simulink model "Woodward_v6_milestone"  (Simulink 7.8)
settings: Solver=ode5  StartTime=0.0  StopTime=inf  FixedStep=Ts  MaxStep=1e-3  RelTol=1e-3
PostLoadFcn:
  | Ts=50e-6;
InitFcn:
  | Ts=50e-6;
undefined symbols (not defined in the file): another_event_name, dfilt, DiscIntNeverNeededParam, fdesignblkfcn, gcbh, Gen_900kW_external_control, GenSet_900kW_07232015, HIL_GenSet, Left, my_event_name, ph, type, V
libraries: simulink x49, powerlib x33, rtio_opalrt_common x19, powerlib_extras x8, dspsigops x4, rtlab x3, cables_lib x3, simulink_extras x3, discretizing x2, rteventslib x2, dsparch4 x2, transformer_lib x1
(part 1 of 3)
settings Model: ARTEMISmethode_block_infos=$$__separator__$$  Creator=CH24070  LastModifiedBy=ma25949  BufferReuse=off
settings SolverCC: ZeroCrossAlgorithm=Adaptive
settings DataIOCC: ExternalInput=getinputstruct(op_snapshot1)  InitialState=getstatestruct(op_snapshot1)  LimitDataPoints=off  MaxDataPoints=90060  SignalLoggingSaveFormat=Dataset  SaveOutput=off  SignalLogging=off  DSMLogging=off  SaveTime=off  OutputSaveName=result
settings OptimizationCC: BlockReduction=off  OptimizeBlockIOStorage=off  BufferReuse=off  ExpressionFolding=off  LocalBlockOutputs=off
settings DebuggingCC: MaxConsecutiveZCsMsg=warning  IgnoredZcDiagnostic=none  SolverPrmCheckMsg=none  MultiTaskRateTransMsg=warning  FrameProcessingCompatibilityMsg=error  ModelReferenceExtraNoncontSigs=warning
settings ModelReferenceCC: UpdateModelReferenceTargets=IfOutOfDate
settings SFSimCC: SFSimEcho=off
settings CodeAppCC: CustomSymbolStrType=$N$R$M_T
settings GRTTargetCC: TargetFunctionLibrary=C89/C90 (ANSI)
settings CustomProperty: DataType=string  Value=0

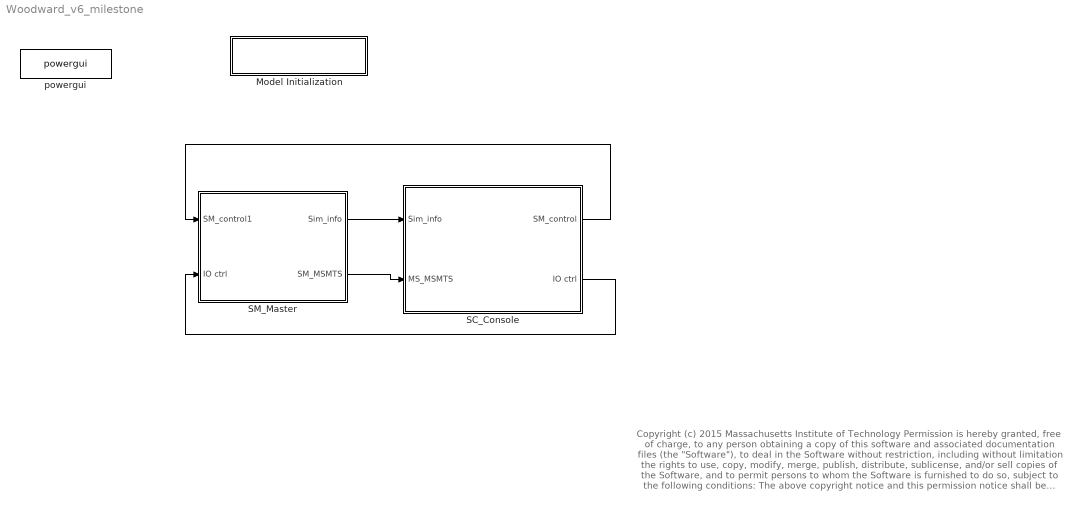
== system Woodward_v6_milestone ==
  note: Copyright (c) 2015 Massachusetts Institute of Technology
      | Permission is hereby granted, free of charge, to any person obtaining a copy of this software and associated documentation files (the "Software"), to deal in the Software without restriction, including without limitation the rights to use, copy, modify, merge, publish, distribute, sublicense, and/or sell copies of the Software, and to permit persons to whom the Software is furnished to do so, subject to the following conditions:
      |
      | The above copyright notice and this permission notice shall be included in all copies or substantial portions of the Software.
      |
      | THE SOFTWARE IS PROVIDED "AS IS", WITHOUT WARRANTY OF ANY KIND, EXPRESS OR IMPLIED, INCLUDING BUT NOT LIMITED TO THE WARRANTIES OF MERCHANTABILITY, FITNESS FOR A PARTICULAR PURPOSE AND NONINFRINGEMENT. IN NO EVENT SHALL THE AUTHORS OR COPYRIGHT HOLDERS BE LIABLE FOR ANY CLAIM,
      | DAMAGES OR OTHER LIABILITY, WHETHER IN AN ACTION OF CONTRACT, TORT OR OTHERWISE, ARISING FROM, OUT OF OR IN CONNECTION WITH THE SOFTWARE OR THE USE OR OTHER DEALINGS IN THE SOFTWARE.
  Model Initialization : Subsystem  AncestorBlock=artemis/Tools /Misc/Model Initialization  mask(Model Functions){InitFcnX=Ts=50e-6;, prel=off, posl=on, inif=on, strf=off}
      mask prompts: InitFcnX "Initialisation"; prel "Preload Function"; posl "PostLoad Function"; inif "InitFcn"; strf "StartFcn"
      mask init:
      | currentBlock = gcb;
      | root = bdroot(currentBlock);
      | 
      | if ~strcmp(get_param(root,'BlockDiagramType'),'library')
      |     if prel==1
      |         set_param(root, 'PreLoadFcn', InitFcnX);
      |     else
      |         set_param(root, 'PreLoadFcn', '');
      |     end
      |     if inif==1
      |         set_param(root, 'InitFcn', InitFcnX);
      |     else
      |         set_param(root, 'InitFcn', '');
      |     end
      |     if strf==1
      |         set_param(root, 'StartFcn', InitFcnX);
      |     else
      |         set_param(root, 'StartFcn', '');
      |     end
      |     if posl==1
      |         set_param(root, 'PostLoadFcn', InitFcnX);
      |     else
      |         set_param(root, 'PostLoadFcn', '');
      |     end
      | end
      | 
      | pos = get_param(currentBlock, 'Position');
      | width = pos(3) - pos(1); height = pos(4) - pos(2);
      | txt = [ upper(root) '\n' '- InitFcn. . . . . '  get_param(root, 'InitFcn') ];
      settings: CopyFcn=set_param(gcb,'LinkStatus','inactive')
      mask Display: text(5, height*0.5, txt, 'horizontalAlignment', 'left', 'verticalAlignment', 'middle') ;
  SC_Console : Subsystem
  SM_Master : Subsystem
  powergui : powerlib/powergui  Priority=2  SimulationMode=Discrete  SolverType=Tustin  SampleTime=Ts  frequency=60  SPID=off  DisableSnubberDevices=off  DisableRonSwitches=off  DisableVfSwitches=off  SwTol=0  Interpol=off  DisplayEquations=off  FunctionMessages=off  frequencyindice=0  Pbase=100e6  ErrMax=1e-4  Iterations=50  UnitsV=kV  UnitsW=MW  echomessages=off  HookPort=off  EnableUseOfTLC=off  x0status=blocks  RestoreLinks=warning  ResistiveCurrentMeasurement=off  Frange=logspace(0,3,50)  Ylog=off  Xlog=off  ShowGrid=off  save=off  variable=ZData  structure=0  ZoomFFT=on  StartTime=0.0  cycles=2  DisplayStyle=off  fundamental=60  FreqAxis=off  MaxFrequency=1000  frequencyindicesteady=1  RmsSteady=1  display=off  Ts=0  methode=off
  wires:
  SM_Master/1(Sim_info) -> SC_Console/1(Sim_info)
  SM_Master/2(SM_MSMTS) -> SC_Console/2(MS_MSMTS)
  SC_Console/1(SM_control) -> SM_Master/1(SM_control1)
  SC_Console/2(IO ctrl) -> SM_Master/2(IO ctrl)

== system Woodward_v6_milestone/Model Initialization ==

== system Woodward_v6_milestone/SC_Console ==
  note: Tcomputation
      | Ttotal
      | Idle
      | Overruns
  note: The 'Overruns' value should remain at 0.
      | The 'Ttotal' value should be equal to the
      | model Fixed-Step size.
  note: Ctrl Error
  Sim_info : Inport
  MS_MSMTS : Inport  Port=2
  B001 : Subsystem
  B031 : Subsystem
  Bus Creator : BusCreator  Inputs=2
  Bus Selector : BusSelector  OutputSignals=B031_PRM,B021_PRM,GEN_900kW_PRM,B012_PRM,B001_PRM,GEN_3p5MW_PRM,signal7,signal8,signal9,Load
  Demux5 : Demux  Outputs=[1 8 4]
  GEN900KW : Subsystem
  Gen_900kW_B001 : Subsystem  AncestorBlock=HIL_GenSet/Gen_900kW_external_control
  Load : Subsystem
  OpComm : rtlab/OpComm  nbport=2  groupe_acq=1  subsys_rate=0  st=0  Synchronization=on  Interpolation=on  Threshold=1.0  Missed_Data=off  Sim_Time=off  Samples=off  dynSigOut=off  from_console=0  warning_done=off  writeOpCommFile=off  Offset=off
  Status Codes : Display
      settings: Decimation=100
  TimingValues : Display
      settings: Decimation=100
  Woodward 900kW : Subsystem
  SM_control : Outport
  IO ctrl : Outport  Port=2
  wires:
  Sim_info/1 -> OpComm/1
  MS_MSMTS/1 -> OpComm/2
  Gen_900kW_B001/1(S) -> Bus Creator/1  "Gen_B001"
  Bus Creator/1 -> SM_control/1
  OpComm/2 -> Bus Selector/1
  Bus Selector/1 -> B031/1(S)  "<B031_PRM>"
  Bus Selector/3 -> GEN900KW/1(S)  "<GEN_900kW_PRM>"
  Bus Selector/5 -> B001/1(S)  "<B001_PRM>"
  Demux5/3 -> TimingValues/1
  OpComm/1 -> Demux5/1
  Demux5/1 -> Status Codes/1
  Bus Selector/8 -> Woodward 900kW/1(Gen_Primary)  "<signal8>"
  Bus Selector/9 -> Woodward 900kW/2(DIn_Ch00_31)  "<signal9>"
  Bus Selector/10 -> Load/1(S)  "<Load>"
  Woodward 900kW/1(Out1) -> IO ctrl/1

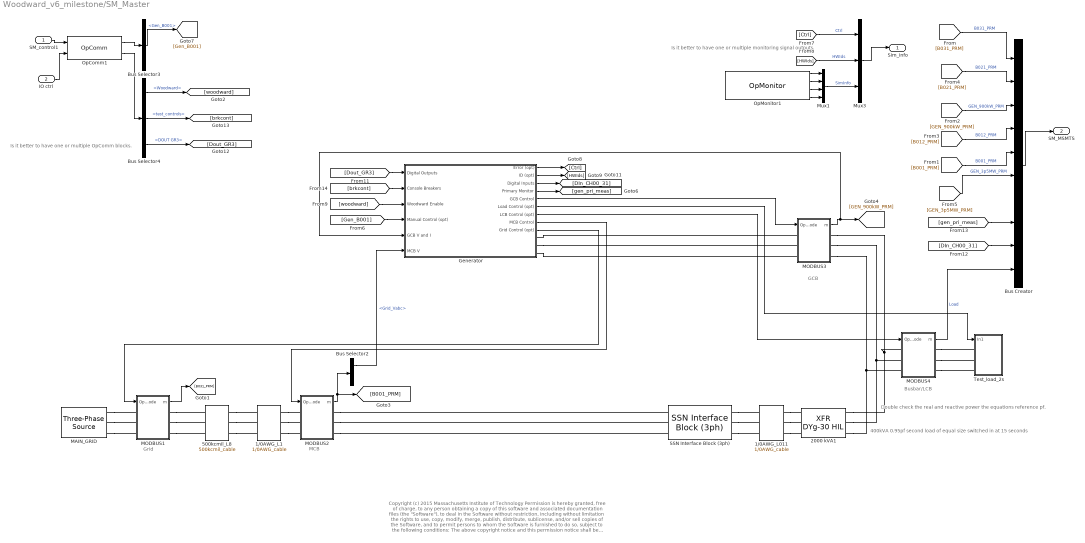
== system Woodward_v6_milestone/SM_Master ==
  note: Double check the real and reactive power
      | the equations reference pf.
  note: 400kVA 0.95pf
      | second load of equal size
      | switched in at 15 seconds
  note: Is it better to have one
      | or multiple OpComm blocks.
  note: Is it better to have one or multiple
      | monitoring signal outputs.
  note: GCB
  note: Busbar/LCB
  note: MCB
  note: Grid
  note: Copyright (c) 2015 Massachusetts Institute of Technology
      | Permission is hereby granted, free of charge, to any person obtaining a copy of this software and associated documentation files (the "Software"), to deal in the Software without restriction, including without limitation the rights to use, copy, modify, merge, publish, distribute, sublicense, and/or sell copies of the Software, and to permit persons to whom the Software is furnished to do so, subject to the following conditions:
      |
      | The above copyright notice and this permission notice shall be included in all copies or substantial portions of the Software.
      |
      | THE SOFTWARE IS PROVIDED "AS IS", WITHOUT WARRANTY OF ANY KIND, EXPRESS OR IMPLIED, INCLUDING BUT NOT LIMITED TO THE WARRANTIES OF MERCHANTABILITY, FITNESS FOR A PARTICULAR PURPOSE AND NONINFRINGEMENT. IN NO EVENT SHALL THE AUTHORS OR COPYRIGHT HOLDERS BE LIABLE FOR ANY CLAIM,
      | DAMAGES OR OTHER LIABILITY, WHETHER IN AN ACTION OF CONTRACT, TORT OR OTHERWISE, ARISING FROM, OUT OF OR IN CONNECTION WITH THE SOFTWARE OR THE USE OR OTHER DEALINGS IN THE SOFTWARE.
  SM_control1 : Inport
  IO ctrl : Inport  Port=2
  1/0AWG_L011 : cables_lib/1//0AWG_cable  length=1000  par_sets=1
  1/0AWG_L1 : cables_lib/1//0AWG_cable  length=1  par_sets=1
  2000 kVA1 : transformer_lib/XFR DYg-30 HIL  Rating=2000  Vp=13800  Vs=480  Z=5.75  XR=5.7
  500kcmil_L8 : cables_lib/500kcmil_cable  length=1  par_sets=1
  Bus Creator : BusCreator  Inputs=10
  Bus Selector2 : BusSelector  OutputSignals=sel_787.Grid_Vabc,sel_787.Iabc
  Bus Selector3 : BusSelector  OutputSignals=Gen_B001
  Bus Selector4 : BusSelector  OutputSignals=Woodward,test_controls,DOUT GR3
  Generator : Subsystem
  MAIN_GRID : powerlib/Electrical Sources/Three-Phase Source  Voltage=13800  PhaseAngle=0  Frequency=60  InternalConnection=Yg  SpecifyImpedance=on  Resistance=0.8929  Inductance=16.58e-3  ShortCircuitLevel=375e6  BaseVoltage=13800  XRratio=7.9  BusType=swing  Pref=0  Qref=0  Qmin=-inf  Qmax=inf
  MODBUS1 : Subsystem  mask(Protection and Metering){IOC=15E3, TOC=1800, Ts=Ts, VRMSLL=13800, I_nom=200}
      mask prompts: IOC "IOC setting [A]"; TOC "TOC setting [A]"; Ts "Sampling Time [Sec]"; VRMSLL "Nominal Voltage [VRMSLL]"; I_nom "Continous Current [A]"
      mask help:
      | This block simulates the behavior of selected relay functions as well as metering equipment.
      | The block is intended to communicate with a microgrid controller providing it measurements, and switching controls.
      mask Help:
      | This block simulates the behavior of selected relay functions as well as metering equipment (60 Hz - only).
      | The block is intended to communicate with a microgrid controller providing it measurements, and switching controls.
      | 
      | The input parameters are:
      | 0) Ts:  Sampling time [Seconds]
      | 1) State: 0 for relay logic mode, 1 to close the controlled breaker/switch,
      | and 2 to open the controlled breaker/switch
      | 2) TOC: Time-inverse overcurrent setting [Amperes]
      | 3) IOC: Instantaneous overcurrent setting [Amperes]
      | 
      | Metered parameters are:
      | 0) Status (0-closed, 1-open)
      | 1) Instantaneous voltage (abc)
      | 2) Instantaneous current (abc)
  MODBUS2 : Subsystem  mask(Protection and Metering){IOC=15E3, TOC=1800, Ts=Ts, VRMSLL=13800, I_nom=200}
      mask prompts: IOC "IOC setting [A]"; TOC "TOC setting [A]"; Ts "Sampling Time [Sec]"; VRMSLL "Nominal Voltage [VRMSLL]"; I_nom "Continous Current [A]"
      mask help:
      | This block simulates the behavior of selected relay functions as well as metering equipment.
      | The block is intended to communicate with a microgrid controller providing it measurements, and switching controls.
      mask Help:
      | This block simulates the behavior of selected relay functions as well as metering equipment (60 Hz - only).
      | The block is intended to communicate with a microgrid controller providing it measurements, and switching controls.
      | 
      | The input parameters are:
      | 0) Ts:  Sampling time [Seconds]
      | 1) State: 0 for relay logic mode, 1 to close the controlled breaker/switch,
      | and 2 to open the controlled breaker/switch
      | 2) TOC: Time-inverse overcurrent setting [Amperes]
      | 3) IOC: Instantaneous overcurrent setting [Amperes]
      | 
      | Metered parameters are:
      | 0) Status (0-closed, 1-open)
      | 1) Instantaneous voltage (abc)
      | 2) Instantaneous current (abc)
  MODBUS3 : Subsystem  mask(Protection and Metering){IOC=15E3, TOC=1800, Ts=Ts, VRMSLL=460, I_nom=200}
      mask prompts: IOC "IOC setting [A]"; TOC "TOC setting [A]"; Ts "Sampling Time [Sec]"; VRMSLL "Nominal Voltage [VRMSLL]"; I_nom "Continous Current [A]"
      mask help:
      | This block simulates the behavior of selected relay functions as well as metering equipment.
      | The block is intended to communicate with a microgrid controller providing it measurements, and switching controls.
      mask Help:
      | This block simulates the behavior of selected relay functions as well as metering equipment (60 Hz - only).
      | The block is intended to communicate with a microgrid controller providing it measurements, and switching controls.
      | 
      | The input parameters are:
      | 0) Ts:  Sampling time [Seconds]
      | 1) State: 0 for relay logic mode, 1 to close the controlled breaker/switch,
      | and 2 to open the controlled breaker/switch
      | 2) TOC: Time-inverse overcurrent setting [Amperes]
      | 3) IOC: Instantaneous overcurrent setting [Amperes]
      | 
      | Metered parameters are:
      | 0) Status (0-closed, 1-open)
      | 1) Instantaneous voltage (abc)
      | 2) Instantaneous current (abc)
  MODBUS4 : Subsystem  mask(Protection and Metering){IOC=15E3, TOC=1800, Ts=Ts, VRMSLL=460, I_nom=200}
      mask prompts: IOC "IOC setting [A]"; TOC "TOC setting [A]"; Ts "Sampling Time [Sec]"; VRMSLL "Nominal Voltage [VRMSLL]"; I_nom "Continous Current [A]"
      mask help:
      | This block simulates the behavior of selected relay functions as well as metering equipment.
      | The block is intended to communicate with a microgrid controller providing it measurements, and switching controls.
      mask Help:
      | This block simulates the behavior of selected relay functions as well as metering equipment (60 Hz - only).
      | The block is intended to communicate with a microgrid controller providing it measurements, and switching controls.
      | 
      | The input parameters are:
      | 0) Ts:  Sampling time [Seconds]
      | 1) State: 0 for relay logic mode, 1 to close the controlled breaker/switch,
      | and 2 to open the controlled breaker/switch
      | 2) TOC: Time-inverse overcurrent setting [Amperes]
      | 3) IOC: Instantaneous overcurrent setting [Amperes]
      | 
      | Metered parameters are:
      | 0) Status (0-closed, 1-open)
      | 1) Instantaneous voltage (abc)
      | 2) Instantaneous current (abc)
  Mux1 : Mux
  Mux3 : Mux  Inputs=[1 8 4]
  OpComm1 : rtlab/OpComm  nbport=2  groupe_acq=1  subsys_rate=0  st=0  Synchronization=on  Interpolation=on  Threshold=1.0  Missed_Data=off  Sim_Time=off  Samples=off  dynSigOut=off  from_console=1  warning_done=off  writeOpCommFile=off  Offset=off
  OpMonitor1 : rtlab/Monitoring/OpMonitor  compute_time=on  real_step=on  idle_time=on  nb_overruns=on  user_time=off  user_name=my_event_name,another_event_name
  SSN Interface Block (3ph) : ssn_lib/SSN Interface Block (3ph)  nb_phase=3  nb_port=2  p1_type=V-type(Left)  p2_type=V-type (Right)  p3_type=V-type(Left)  p4_type=V-type(Left)  p5_type=V-type(Left)  p6_type=V-type(Left)  p7_type=V-type(Left)  p8_type=V-type(Left)  p9_type=V-type(Left)  p10_type=V-type(Left)  p11_type=V-type(Left)  p12_type=V-type(Left)  p13_type=V-type(Left)  p14_type=V-type(Left)  p15_type=V-type(Left)  p16_type=V-type(Left)  I_port_shunt_resistance=1e9
  Test_load_2s : Subsystem  mask{v=460, kVA=400, pf=0.95}
      mask prompts: v "VRMSLL"
  Sim_info : Outport
  SM_MSMTS : Outport  Port=2
  wires:
  [B031_PRM] -> Bus Creator/1  "B031_PRM"
  [GEN_900kW_PRM] -> Bus Creator/3  "GEN_900kW_PRM"
  [B012_PRM] -> Bus Creator/4  "B012_PRM"
  [B021_PRM] -> Bus Creator/2  "B021_PRM"
  Bus Creator/1 -> SM_MSMTS/1
  [B001_PRM] -> Bus Creator/5  "B001_PRM"
  [GEN_3p5MW_PRM] -> Bus Creator/6  "GEN_3p5MW_PRM"
  [DIn_CH00_31] -> Bus Creator/9
  SM_control1/1 -> OpComm1/1
  OpComm1/1 -> Bus Selector3/1
  Bus Selector3/1 -> [Gen_B001]  "<Gen_B001>"
  OpComm1/2 -> Bus Selector4/1
  Bus Selector4/1 -> [woodward]  "<Woodward>"
  IO ctrl/1 -> OpComm1/2
  Bus Selector4/3 -> [Dout_GR3]  "<DOUT GR3>"
  OpMonitor1/1 -> Mux1/1
  OpMonitor1/2 -> Mux1/2
  OpMonitor1/3 -> Mux1/3
  OpMonitor1/4 -> Mux1/4
  Mux1/1 -> Mux3/3  "SimInfo"
  [Ctrl] -> Mux3/1  "Ctrl"
  [HWIds] -> Mux3/2  "HWIds"
  Mux3/1 -> Sim_info/1
  [gen_pri_meas] -> Bus Creator/8
  Bus Selector4/2 -> [brkcont]  "<test_controls>"
  MODBUS1/1(m) -> [B031_PRM]
  MODBUS2/1(m) -> Bus Selector2/1, [B001_PRM]
  MODBUS3/1(m) -> [GEN_900kW_PRM], Generator/5(GCB V and I)
  MODBUS4/1(m) -> Bus Creator/10  "Load"
  [Dout_GR3] -> Generator/1(Digital Outputs)
  [brkcont] -> Generator/2(Console Breakers)
  Generator/4(Primary Monitor) -> [gen_pri_meas]
  Generator/1(Error (opt)) -> [Ctrl]
  Generator/2(ID (opt)) -> [HWIds]
  Generator/3(Digital Inputs) -> [DIn_CH00_31]
  Bus Selector2/1 -> Generator/6(MCB V)  "<Grid_Vabc>"
  [Gen_B001] -> Generator/4(Manual Control (opt))
  [woodward] -> Generator/3(Woodward Enable)
  Generator/5(GCB Control) -> MODBUS3/1(Op_Mode)
  Generator/6(Load Control (opt)) -> Test_load_2s/1(In1)
  Generator/7(LCB Control (opt)) -> MODBUS4/1(Op_Mode)
  Generator/8(MCB Control) -> MODBUS2/1(Op_Mode)
  Generator/9(Grid Control (opt)) -> MODBUS1/1(Op_Mode)
  connections:
  1/0AWG_L011/RConn1 -- 2000 kVA1/LConn1
  1/0AWG_L011/RConn2 -- 2000 kVA1/LConn2
  1/0AWG_L011/RConn3 -- 2000 kVA1/LConn3
  SSN Interface Block (3ph)/RConn3 -- 1/0AWG_L011/LConn3
  SSN Interface Block (3ph)/RConn2 -- 1/0AWG_L011/LConn2
  SSN Interface Block (3ph)/RConn1 -- 1/0AWG_L011/LConn1
  MODBUS4/RConn3 -- Test_load_2s/LConn3
  MODBUS4/RConn2 -- Test_load_2s/LConn2
  MODBUS4/RConn1 -- Test_load_2s/LConn1
  2000 kVA1/RConn3 -- MODBUS4/LConn3 -- MODBUS3/RConn3
  2000 kVA1/RConn2 -- MODBUS4/LConn2 -- MODBUS3/RConn2
  2000 kVA1/RConn1 -- MODBUS4/LConn1 -- MODBUS3/RConn1
  MODBUS1/RConn3 -- 500kcmil_L8/LConn3
  MODBUS1/RConn2 -- 500kcmil_L8/LConn2
  MODBUS1/RConn1 -- 500kcmil_L8/LConn1
  MAIN_GRID/RConn3 -- MODBUS1/LConn3
  MAIN_GRID/RConn2 -- MODBUS1/LConn2
  MAIN_GRID/RConn1 -- MODBUS1/LConn1
  Generator/RConn3 -- MODBUS3/LConn3
  Generator/RConn2 -- MODBUS3/LConn2
  Generator/RConn1 -- MODBUS3/LConn1
  MODBUS2/RConn3 -- SSN Interface Block (3ph)/LConn3
  MODBUS2/RConn2 -- SSN Interface Block (3ph)/LConn2
  MODBUS2/RConn1 -- SSN Interface Block (3ph)/LConn1
  500kcmil_L8/RConn1 -- 1/0AWG_L1/LConn1
  500kcmil_L8/RConn2 -- 1/0AWG_L1/LConn2
  500kcmil_L8/RConn3 -- 1/0AWG_L1/LConn3
  1/0AWG_L1/RConn1 -- MODBUS2/LConn1
  1/0AWG_L1/RConn2 -- MODBUS2/LConn2
  1/0AWG_L1/RConn3 -- MODBUS2/LConn3

== system Woodward_v6_milestone/SC_Console/B001 ==
  S : Inport
  Bus Selector : BusSelector  OutputSignals=Grid_Status,sel_787.Grid_Vabc,sel_787.Iabc,sel_787.Grid_P,sel_787.Grid_Q
  Scope Mains : Scope  NumInputPorts=5
      settings: TimeRange=20  YMin=0~-15000~-500~-1e+006~-1e+006  YMax=1~15000~500~1e+006~1e+006  SaveName=ScopeData6
  wires:
  S/1 -> Bus Selector/1
  Bus Selector/1 -> Scope Mains/1  "<Grid_Status>"
  Bus Selector/2 -> Scope Mains/2  "<Grid_Vabc>"
  Bus Selector/3 -> Scope Mains/3  "<Iabc>"
  Bus Selector/4 -> Scope Mains/4  "<Grid_P>"
  Bus Selector/5 -> Scope Mains/5  "<Grid_Q>"

== system Woodward_v6_milestone/SC_Console/B031 ==
  S : Inport
  Bus Selector : BusSelector  OutputSignals=Grid_Status,sel_787.Grid_Vabc,sel_787.Iabc,sel_787.Grid_P,sel_787.Grid_Q
  Scope Grid : Scope  NumInputPorts=5
      settings: TimeRange=20  YMin=0~-20000~-20000~-1e+006~-1e+006  YMax=1~20000~20000~1e+006~1e+006
  wires:
  Bus Selector/1 -> Scope Grid/1  "<Grid_Status>"
  Bus Selector/2 -> Scope Grid/2  "<Grid_Vabc>"
  Bus Selector/3 -> Scope Grid/3  "<Iabc>"
  Bus Selector/4 -> Scope Grid/4  "<Grid_P>"
  Bus Selector/5 -> Scope Grid/5  "<Grid_Q>"
  S/1 -> Bus Selector/1

== system Woodward_v6_milestone/SC_Console/GEN900KW ==
  S : Inport
  Bus Selector : BusSelector  OutputSignals=Grid_Status,sel_787.Grid_Vabc,sel_787.Iabc,sel_787.Grid_P,sel_787.Grid_Q
  Scope Gen : Scope  NumInputPorts=5
      settings: TimeRange=60  YMin=0~-700~-2000~-1000000~-1000000  YMax=1~700~2000~1000000~1000000  SaveName=ScopeData5
  wires:
  S/1 -> Bus Selector/1
  Bus Selector/1 -> Scope Gen/1  "<Grid_Status>"
  Bus Selector/2 -> Scope Gen/2  "<Grid_Vabc>"
  Bus Selector/3 -> Scope Gen/3  "<Iabc>"
  Bus Selector/4 -> Scope Gen/4  "<Grid_P>"
  Bus Selector/5 -> Scope Gen/5  "<Grid_Q>"

== system Woodward_v6_milestone/SC_Console/Gen_900kW_B001 ==
  1 - PQ 2 - PV 3 - VF : Constant  Value=3
  Bus Creator : BusCreator  Inputs=6
  DONOTCHANGE : Constant
  Enable = 1 Disable = 0 : Constant  Value=0
  F : simulink/Math Operations/Slider Gain  low=0.97  gain=1  high=1.03
  P : simulink/Math Operations/Slider Gain  low=0  gain=0.8  high=1.1
  Q : simulink/Math Operations/Slider Gain  low=0.01  gain=0.2  high=0.4
  V : simulink/Math Operations/Slider Gain  low=0.9  gain=1  high=1.1
  S : Outport
  wires:
  DONOTCHANGE/1 -> P/1, Q/1, V/1, F/1
  Bus Creator/1 -> S/1
  P/1 -> Bus Creator/1  "P"
  Q/1 -> Bus Creator/2  "Q"
  V/1 -> Bus Creator/3  "V"
  F/1 -> Bus Creator/4  "F"
  1 - PQ 2 - PV 3 - VF/1 -> Bus Creator/5  "Mode"
  Enable = 1 Disable = 0/1 -> Bus Creator/6  "Enable"

== system Woodward_v6_milestone/SC_Console/Load ==
  S : Inport
  Bus Selector : BusSelector  OutputSignals=Grid_Status,sel_787.Grid_Vabc,sel_787.Iabc,sel_787.Grid_P,sel_787.Grid_Q
  Scope Load : Scope  NumInputPorts=5
      settings: TimeRange=20  YMin=0~-600~-2000~-1e+006~-1e+006  YMax=1~600~2000~1e+006~1e+006
  wires:
  Bus Selector/1 -> Scope Load/1  "<Grid_Status>"
  Bus Selector/2 -> Scope Load/2  "<Grid_Vabc>"
  Bus Selector/3 -> Scope Load/3  "<Iabc>"
  Bus Selector/4 -> Scope Load/4  "<Grid_P>"
  Bus Selector/5 -> Scope Load/5  "<Grid_Q>"
  S/1 -> Bus Selector/1

== system Woodward_v6_milestone/SC_Console/Woodward 900kW ==
  note: Op_Mode:
      | 0 = Relay Functions
      | 1 = Close Breaker
      | 2 = Open Breaker
  note: This corresponds to
      | the DIO Enable MCB
  Gen_Primary : Inport
  DIn_Ch00_31 : Inport  Port=2
  16Din/16Dout GR3 : Subsystem
  16PWMIn/16PWMout GR3 : Subsystem
  16TSDIn/16 TSDOut GR3 : Subsystem
  Brk1 Grid : Constant  Value=2
  Brk2 MCB : Constant  Value=2
  Brk3 GCB : Constant
  Brk4 Load : Constant  Value=2
  Bus Creator1 : BusCreator  Inputs=3
  Bus Creator2 : BusCreator  Inputs=3
  Bus Creator3 : BusCreator  Inputs=9
  Bus Selector1 : BusSelector  OutputSignals=Pm,Vf,Vt,w
  Scope_Primary : Scope  NumInputPorts=4
      settings: TimeRange=60  YMin=0~-5~-1~-1  YMax=1.1~5~2~2  SaveName=ScopeData4
  Wood MCB Enable : Constant  Value=0
  bias_ctrl : Constant
  control mode 1 for Woodward 0 for simulation 1 : Constant
  control_mode : Constant
  gen_enable : Constant  Value=0
  load mode 1 for add load 0 for no added load : Constant  Value=0
  Out1 : Outport
  wires:
  control mode 1 for Woodward 0 for simulation 1/1 -> Bus Creator2/1  "Woodward"
  16Din/16Dout GR3/1(Dout) -> Bus Creator1/1  "16 DOUT GR3"
  16TSDIn/16 TSDOut GR3/1(TSDout) -> Bus Creator1/2  "16 TSDOUT GR3"
  16PWMIn/16PWMout GR3/1(To PWMOut) -> Bus Creator1/3  "16 PWMOUT GR3"
  Bus Creator1/1 -> Bus Creator2/3  "DOUT GR3"
  Bus Creator3/1 -> Bus Creator2/2  "test_controls"
  Brk1 Grid/1 -> Bus Creator3/1  "Grid"
  Brk2 MCB/1 -> Bus Creator3/2  "MCB"
  Brk3 GCB/1 -> Bus Creator3/3  "GCB"
  Brk4 Load/1 -> Bus Creator3/4  "LCB"
  load mode 1 for add load 0 for no added load/1 -> Bus Creator3/5  "Load"
  control_mode/1 -> Bus Creator3/6  "Wood_DIO"
  gen_enable/1 -> Bus Creator3/7  "Gen_enable"
  bias_ctrl/1 -> Bus Creator3/8  "Gen_bias_enable"
  Bus Creator2/1 -> Out1/1
  DIn_Ch00_31/1 -> 16Din/16Dout GR3/1(Din)
  Bus Selector1/1 -> Scope_Primary/1  "<Pm>"
  Bus Selector1/2 -> Scope_Primary/2  "<Vf>"
  Bus Selector1/3 -> Scope_Primary/3  "<Vt>"
  Bus Selector1/4 -> Scope_Primary/4  "<w>"
  Gen_Primary/1 -> Bus Selector1/1
  Wood MCB Enable/1 -> Bus Creator3/9  "Wood_MCB_enable"

== system Woodward_v6_milestone/SM_Master/Generator ==
  note: The woodward is set to VF mode the entire time.
  note: Op_Mode:
      | 0 = Relay Functions
      | 1 = Close Breaker
      | 2 = Open Breaker
  Digital Outputs : Inport
  Console Breakers : Inport  Port=2
  Woodward Enable : Inport  Port=3
  Manual Control (opt) : Inport  Port=4
  GCB V and I : Inport  Port=5
  MCB V : Inport  Port=6
  Bus Selector5 : BusSelector  OutputSignals=Wood_DIO,Gen_bias_enable,Gen_enable,GCB,Load,LCB,Wood_MCB_enable,MCB,Grid
  Bus Selector6 : BusSelector  OutputSignals=sel_787.Grid_Vabc,sel_787.Iabc
  Bus Selector7 : BusSelector  OutputSignals="w.w.Rotor speed  wm (pu)"
  GenSet_900kW_07232015 : Subsystem  AncestorBlock=HIL_GenSet/GenSet_900kW_07232015  mask(Gen-Set with simulated control modes){control_mode=1}
      mask prompts: control_mode "Control Mode [0 => Sim. 1 => Wood.]"
      mask help:
      | This Gen-Set block allows the user to indicate the control mode of the generator. The available control modes are: (1) PQ, (2) PV, and (3) VF.
      | The input values to the block will be applied according to the selected control mode.
      | For example, if PQ mode is selected, the controller will only work based on P_ref and Q_ref ignoring values of other inputs to the block.
  Switch : Switch  Threshold=0.5
  Woodward Inputs : Subsystem
  Woodward Outputs : Subsystem
  A : PMIOPort  Port=1  Side=Right
  B : PMIOPort  Port=2  Side=Right
  C : PMIOPort  Port=3  Side=Right
  Error (opt) : Outport
  ID (opt) : Outport  Port=2
  Digital Inputs : Outport  Port=3
  Primary Monitor : Outport  Port=4
  GCB Control : Outport  Port=5
  Load Control (opt) : Outport  Port=6
  LCB Control (opt) : Outport  Port=7
  MCB Control : Outport  Port=8
  Grid Control (opt) : Outport  Port=9
  wires:
  GenSet_900kW_07232015/1(gen_primary) -> Bus Selector7/1, Primary Monitor/1
  Bus Selector6/1 -> Woodward Inputs/2(Generator_Voltage)  "<Grid_Vabc>"
  Bus Selector6/2 -> Woodward Inputs/3(Generator_Current)  "<Iabc>"
  Bus Selector5/1 -> Woodward Outputs/2(DIO Enable)  "<Wood_DIO>"
  Manual Control (opt)/1 -> GenSet_900kW_07232015/7(Manual_control)
  Woodward Outputs/6(GOV) -> GenSet_900kW_07232015/3(Woodward meas w)
  Woodward Outputs/7(AVR) -> GenSet_900kW_07232015/4(Woodward meas V)
  Bus Selector5/2 -> Woodward Outputs/3(Bias Enable)  "<Gen_bias_enable>"
  Woodward Outputs/4(Ref Gov) -> GenSet_900kW_07232015/1(Woodward Modbus Ref for Governor)
  Woodward Outputs/5(Ref AVR) -> GenSet_900kW_07232015/2(Woodward Modbus Ref for AVR)
  Bus Selector7/1 -> Woodward Inputs/1(MPU_speed)  "<Rotor speed  wm (pu)>"
  Woodward Outputs/1(Error) -> Error (opt)/1
  Woodward Outputs/2(IDs) -> ID (opt)/1
  Woodward Outputs/3(Digital Inputs) -> Digital Inputs/1
  Woodward Enable/1 -> GenSet_900kW_07232015/6(Woodward Enable)
  Woodward Outputs/8(Fuel Enable) -> GenSet_900kW_07232015/5(Generator Enable)
  Bus Selector5/7 -> Switch/2  "<Wood_MCB_enable>"
  Bus Selector5/8 -> Switch/3  "<MCB>"
  Woodward Outputs/10(MCB) -> Switch/1
  Digital Outputs/1 -> Woodward Outputs/1(Digital Output)
  GCB V and I/1 -> Bus Selector6/1
  MCB V/1 -> Woodward Inputs/4(Mains_Voltage)
  Woodward Outputs/9(GCB) -> GCB Control/1
  Console Breakers/1 -> Bus Selector5/1
  Bus Selector5/5 -> Load Control (opt)/1  "<Load>"
  Bus Selector5/6 -> LCB Control (opt)/1  "<LCB>"
  Switch/1 -> MCB Control/1
  Bus Selector5/9 -> Grid Control (opt)/1  "<Grid>"
  connections:
  A/RConn1 -- GenSet_900kW_07232015/RConn1
  B/RConn1 -- GenSet_900kW_07232015/RConn2
  C/RConn1 -- GenSet_900kW_07232015/RConn3

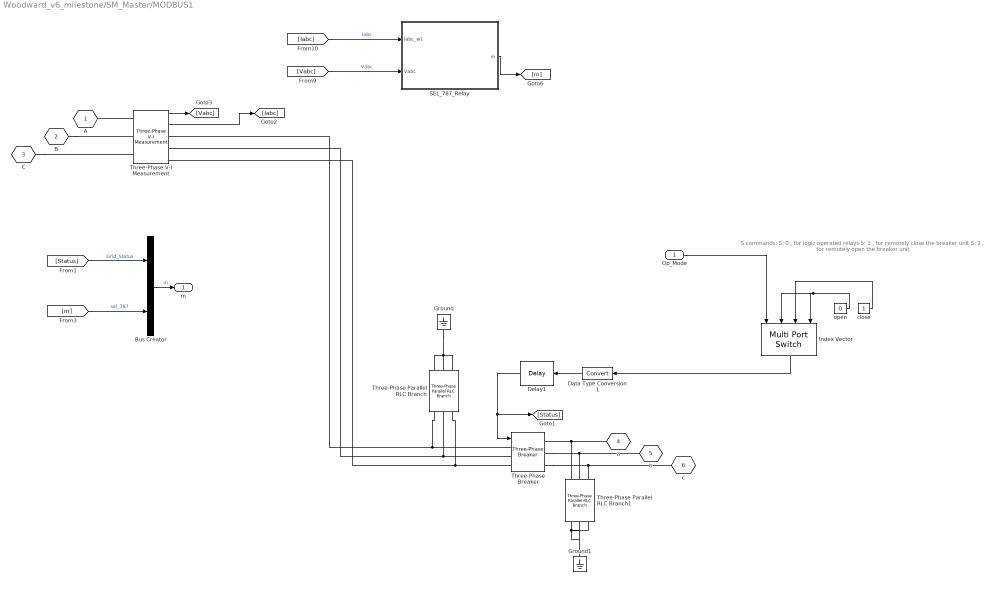
== system Woodward_v6_milestone/SM_Master/MODBUS1 ==
  note: S commands:
      | S: 0 , for logic operated relays
      | S: 1 ,  for remotely close the breaker unit
      | S: 2 , for remotely open the breaker unit
  Op_Mode : Inport
  Bus Creator : BusCreator  Inputs=2
  Data Type Conversion1 : DataTypeConversion
  Delay1 : dspsigops/Delay  dly_unit=Samples  delay=lower((3/60)/Ts)  ic_detail=off  dif_ic_for_ch=off  dif_ic_for_dly=off  ic=1  reset_popup=None
  Ground : powerlib/Elements/Ground  LConnTagsString=a
  Ground1 : powerlib/Elements/Ground  LConnTagsString=a
  Index Vector : MultiPortSwitch  DataPortOrder=Zero-based contiguous  DataPortIndices={2,1,0}  zeroidx=on
  SEL_787_Relay : Subsystem
  Three-Phase Parallel RLC Branch : powerlib/Elements/Three-Phase Parallel RLC Branch  LConnTagsString=A|B|C  RConnTagsString=A|B|C  BranchType=R  Resistance=10e6  Inductance=1e-3  Capacitance=1e-6  Measurements=None
  Three-Phase Parallel RLC Branch1 : powerlib/Elements/Three-Phase Parallel RLC Branch  LConnTagsString=A|B|C  RConnTagsString=A|B|C  BranchType=R  Resistance=10e6  Inductance=1e-3  Capacitance=1e-6  Measurements=None
  Three-Phase V-I Measurement : powerlib/Measurements/Three-Phase V-I Measurement  VoltageMeasurement=phase-to-ground  SetLabelV=off  LabelV=Vabc  Vpu=off  VpuLL=off  CurrentMeasurement=yes  SetLabelI=off  LabelI=Iabc  Ipu=off  Pbase=100e6  Vbase=500e3  OutputType=Complex  PhasorSimulation=off  PSBequivalent=0
  Three-Phase Breaker : powerlib/Elements/Three-Phase Breaker  InitialState=closed  SwitchA=on  SwitchB=on  SwitchC=on  SwitchTimes="[1/60  5/60]"  External=on  BreakerResistance=1e-3  SnubberResistance=0  SnubberCapacitance=0  Measurements=None
  close : Constant
  open : Constant  Value=0
  A : PMIOPort  Tag=PMCPort  Port=1  Side=Left
  B : PMIOPort  Tag=PMCPort  Port=2  Side=Left
  C : PMIOPort  Tag=PMCPort  Port=3  Side=Left
  a : PMIOPort  Tag=PMCPort  Port=4  Side=Right
  b : PMIOPort  Tag=PMCPort  Port=5  Side=Right
  c : PMIOPort  Tag=PMCPort  Port=6  Side=Right
  m : Outport
  wires:
  [m] -> Bus Creator/2  "sel_787"
  SEL_787_Relay/1(m) -> [m]
  Bus Creator/1 -> m/1  "m"
  [Status] -> Bus Creator/1  "Grid_Status"
  Delay1/1 -> [Status], Three-Phase Breaker/1
  Three-Phase V-I Measurement/1 -> [Vabc]
  Three-Phase V-I Measurement/2 -> [Iabc]
  open/1 -> Index Vector/4, Index Vector/2
  close/1 -> Index Vector/3
  Index Vector/1 -> Data Type Conversion1/1
  Data Type Conversion1/1 -> Delay1/1
  [Iabc] -> SEL_787_Relay/1(Iabc_w1)  "Iabc"
  [Vabc] -> SEL_787_Relay/2(Vabc)  "Vabc"
  Op_Mode/1 -> Index Vector/1
  connections:
  Three-Phase Breaker/LConn1 -- Three-Phase V-I Measurement/RConn1 -- Three-Phase Parallel RLC Branch/RConn1
  Three-Phase Breaker/LConn2 -- Three-Phase V-I Measurement/RConn2 -- Three-Phase Parallel RLC Branch/RConn2
  Three-Phase Breaker/LConn3 -- Three-Phase V-I Measurement/RConn3 -- Three-Phase Parallel RLC Branch/RConn3
  Three-Phase Breaker/RConn2 -- b/RConn1 -- Three-Phase Parallel RLC Branch1/RConn2
  Three-Phase Breaker/RConn3 -- c/RConn1 -- Three-Phase Parallel RLC Branch1/RConn3
  Three-Phase V-I Measurement/LConn1 -- A/RConn1
  a/RConn1 -- Three-Phase Breaker/RConn1 -- Three-Phase Parallel RLC Branch1/RConn1
  C/RConn1 -- Three-Phase V-I Measurement/LConn3
  B/RConn1 -- Three-Phase V-I Measurement/LConn2
  Three-Phase Parallel RLC Branch1/LConn1 -- Ground1/LConn1 -- Three-Phase Parallel RLC Branch1/LConn2 -- Three-Phase Parallel RLC Branch1/LConn3
  Ground/LConn1 -- Three-Phase Parallel RLC Branch/LConn2 -- Three-Phase Parallel RLC Branch/LConn3 -- Three-Phase Parallel RLC Branch/LConn1

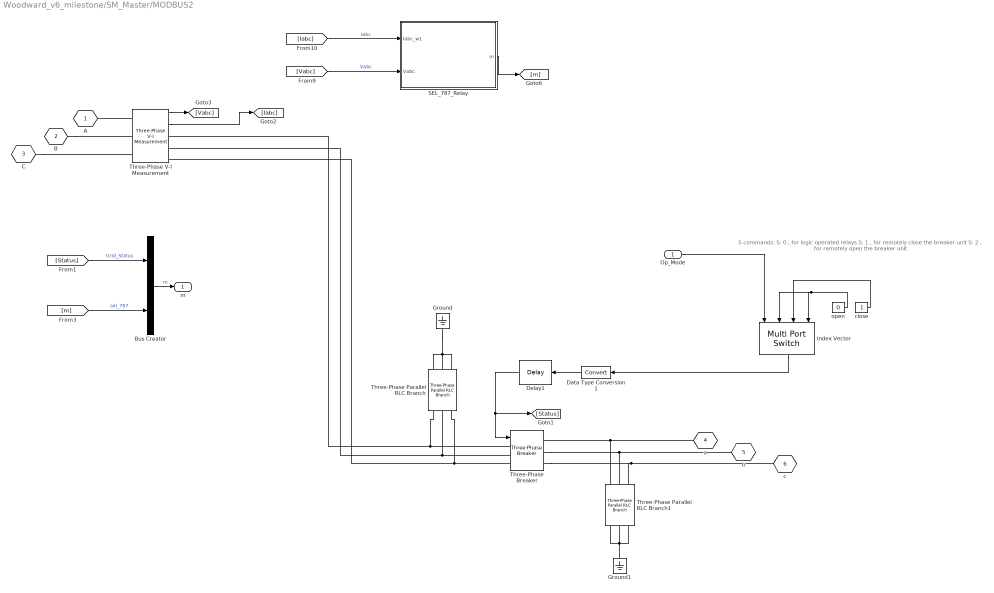
== system Woodward_v6_milestone/SM_Master/MODBUS2 ==
  note: S commands:
      | S: 0 , for logic operated relays
      | S: 1 ,  for remotely close the breaker unit
      | S: 2 , for remotely open the breaker unit
  Op_Mode : Inport
  Bus Creator : BusCreator  Inputs=2
  Data Type Conversion1 : DataTypeConversion
  Delay1 : dspsigops/Delay  dly_unit=Samples  delay=lower((3/60)/Ts)  ic_detail=off  dif_ic_for_ch=off  dif_ic_for_dly=off  ic=1  reset_popup=None
  Ground : powerlib/Elements/Ground  LConnTagsString=a
  Ground1 : powerlib/Elements/Ground  LConnTagsString=a
  Index Vector : MultiPortSwitch  DataPortOrder=Zero-based contiguous  DataPortIndices={2,1,0}  zeroidx=on
  SEL_787_Relay : Subsystem
  Three-Phase Parallel RLC Branch : powerlib/Elements/Three-Phase Parallel RLC Branch  LConnTagsString=A|B|C  RConnTagsString=A|B|C  BranchType=R  Resistance=10e6  Inductance=1e-3  Capacitance=1e-6  Measurements=None
  Three-Phase Parallel RLC Branch1 : powerlib/Elements/Three-Phase Parallel RLC Branch  LConnTagsString=A|B|C  RConnTagsString=A|B|C  BranchType=R  Resistance=10e6  Inductance=1e-3  Capacitance=1e-6  Measurements=None
  Three-Phase V-I Measurement : powerlib/Measurements/Three-Phase V-I Measurement  VoltageMeasurement=phase-to-ground  SetLabelV=off  LabelV=Vabc  Vpu=off  VpuLL=off  CurrentMeasurement=yes  SetLabelI=off  LabelI=Iabc  Ipu=off  Pbase=100e6  Vbase=500e3  OutputType=Complex  PhasorSimulation=off  PSBequivalent=0
  Three-Phase Breaker : powerlib/Elements/Three-Phase Breaker  InitialState=closed  SwitchA=on  SwitchB=on  SwitchC=on  SwitchTimes="[1/60  5/60]"  External=on  BreakerResistance=1e-3  SnubberResistance=0  SnubberCapacitance=0  Measurements=None
  close : Constant
  open : Constant  Value=0
  A : PMIOPort  Tag=PMCPort  Port=1  Side=Left
  B : PMIOPort  Tag=PMCPort  Port=2  Side=Left
  C : PMIOPort  Tag=PMCPort  Port=3  Side=Left
  a : PMIOPort  Tag=PMCPort  Port=4  Side=Right
  b : PMIOPort  Tag=PMCPort  Port=5  Side=Right
  c : PMIOPort  Tag=PMCPort  Port=6  Side=Right
  m : Outport
  wires:
  [m] -> Bus Creator/2  "sel_787"
  SEL_787_Relay/1(m) -> [m]
  Bus Creator/1 -> m/1  "m"
  [Status] -> Bus Creator/1  "Grid_Status"
  Delay1/1 -> [Status], Three-Phase Breaker/1
  Three-Phase V-I Measurement/1 -> [Vabc]
  Three-Phase V-I Measurement/2 -> [Iabc]
  open/1 -> Index Vector/4, Index Vector/2
  close/1 -> Index Vector/3
  Index Vector/1 -> Data Type Conversion1/1
  Data Type Conversion1/1 -> Delay1/1
  [Iabc] -> SEL_787_Relay/1(Iabc_w1)  "Iabc"
  [Vabc] -> SEL_787_Relay/2(Vabc)  "Vabc"
  Op_Mode/1 -> Index Vector/1
  connections:
  Three-Phase V-I Measurement/RConn1 -- Three-Phase Parallel RLC Branch/RConn1 -- Three-Phase Breaker/LConn1
  Three-Phase V-I Measurement/RConn2 -- Three-Phase Parallel RLC Branch/RConn2 -- Three-Phase Breaker/LConn2
  Three-Phase V-I Measurement/RConn3 -- Three-Phase Parallel RLC Branch/RConn3 -- Three-Phase Breaker/LConn3
  Three-Phase Breaker/RConn2 -- b/RConn1 -- Three-Phase Parallel RLC Branch1/RConn2
  Three-Phase Breaker/RConn3 -- c/RConn1 -- Three-Phase Parallel RLC Branch1/RConn3
  Three-Phase V-I Measurement/LConn1 -- A/RConn1
  a/RConn1 -- Three-Phase Breaker/RConn1 -- Three-Phase Parallel RLC Branch1/RConn1
  C/RConn1 -- Three-Phase V-I Measurement/LConn3
  B/RConn1 -- Three-Phase V-I Measurement/LConn2
  Ground/LConn1 -- Three-Phase Parallel RLC Branch/LConn2 -- Three-Phase Parallel RLC Branch/LConn3 -- Three-Phase Parallel RLC Branch/LConn1
  Three-Phase Parallel RLC Branch1/LConn1 -- Ground1/LConn1 -- Three-Phase Parallel RLC Branch1/LConn2 -- Three-Phase Parallel RLC Branch1/LConn3

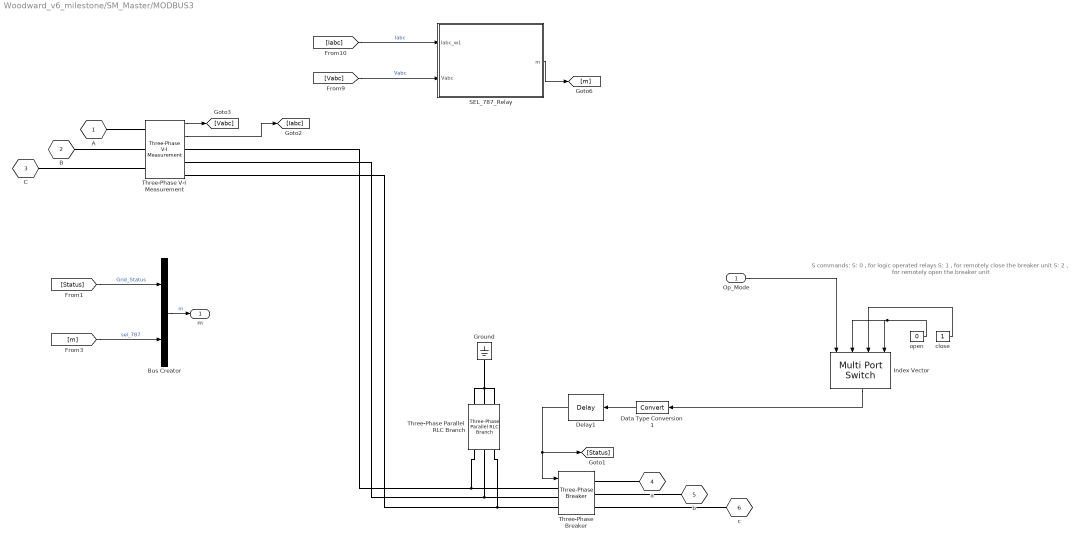
== system Woodward_v6_milestone/SM_Master/MODBUS3 ==
  note: S commands:
      | S: 0 , for logic operated relays
      | S: 1 ,  for remotely close the breaker unit
      | S: 2 , for remotely open the breaker unit
  Op_Mode : Inport
  Bus Creator : BusCreator  Inputs=2
  Data Type Conversion1 : DataTypeConversion
  Delay1 : dspsigops/Delay  dly_unit=Samples  delay=lower((3/60)/Ts)  ic_detail=off  dif_ic_for_ch=off  dif_ic_for_dly=off  ic=1  reset_popup=None
  Ground : powerlib/Elements/Ground  LConnTagsString=a
  Index Vector : MultiPortSwitch  DataPortOrder=Zero-based contiguous  DataPortIndices={2,1,0}  zeroidx=on
  SEL_787_Relay : Subsystem
  Three-Phase Parallel RLC Branch : powerlib/Elements/Three-Phase Parallel RLC Branch  LConnTagsString=A|B|C  RConnTagsString=A|B|C  BranchType=R  Resistance=10e6  Inductance=1e-3  Capacitance=1e-6  Measurements=None
  Three-Phase V-I Measurement : powerlib/Measurements/Three-Phase V-I Measurement  VoltageMeasurement=phase-to-ground  SetLabelV=off  LabelV=Vabc  Vpu=off  VpuLL=off  CurrentMeasurement=yes  SetLabelI=off  LabelI=Iabc  Ipu=off  Pbase=100e6  Vbase=500e3  OutputType=Complex  PhasorSimulation=off  PSBequivalent=0
  Three-Phase Breaker : powerlib/Elements/Three-Phase Breaker  InitialState=closed  SwitchA=on  SwitchB=on  SwitchC=on  SwitchTimes="[1/60  5/60]"  External=on  BreakerResistance=1e-3  SnubberResistance=0  SnubberCapacitance=0  Measurements=None
  close : Constant
  open : Constant  Value=0
  A : PMIOPort  Tag=PMCPort  Port=1  Side=Left
  B : PMIOPort  Tag=PMCPort  Port=2  Side=Left
  C : PMIOPort  Tag=PMCPort  Port=3  Side=Left
  a : PMIOPort  Tag=PMCPort  Port=4  Side=Right
  b : PMIOPort  Tag=PMCPort  Port=5  Side=Right
  c : PMIOPort  Tag=PMCPort  Port=6  Side=Right
  m : Outport
  wires:
  [m] -> Bus Creator/2  "sel_787"
  SEL_787_Relay/1(m) -> [m]
  Bus Creator/1 -> m/1  "m"
  [Status] -> Bus Creator/1  "Grid_Status"
  Delay1/1 -> [Status], Three-Phase Breaker/1
  Three-Phase V-I Measurement/1 -> [Vabc]
  Three-Phase V-I Measurement/2 -> [Iabc]
  open/1 -> Index Vector/4, Index Vector/2
  close/1 -> Index Vector/3
  Index Vector/1 -> Data Type Conversion1/1
  Data Type Conversion1/1 -> Delay1/1
  [Iabc] -> SEL_787_Relay/1(Iabc_w1)  "Iabc"
  [Vabc] -> SEL_787_Relay/2(Vabc)  "Vabc"
  Op_Mode/1 -> Index Vector/1
  connections:
  Three-Phase V-I Measurement/RConn1 -- Three-Phase Parallel RLC Branch/RConn1 -- Three-Phase Breaker/LConn1
  Three-Phase V-I Measurement/RConn2 -- Three-Phase Parallel RLC Branch/RConn2 -- Three-Phase Breaker/LConn2
  Three-Phase V-I Measurement/RConn3 -- Three-Phase Parallel RLC Branch/RConn3 -- Three-Phase Breaker/LConn3
  Three-Phase Breaker/RConn2 -- b/RConn1
  Three-Phase Breaker/RConn3 -- c/RConn1
  Three-Phase V-I Measurement/LConn1 -- A/RConn1
  a/RConn1 -- Three-Phase Breaker/RConn1
  C/RConn1 -- Three-Phase V-I Measurement/LConn3
  B/RConn1 -- Three-Phase V-I Measurement/LConn2
  Ground/LConn1 -- Three-Phase Parallel RLC Branch/LConn2 -- Three-Phase Parallel RLC Branch/LConn3 -- Three-Phase Parallel RLC Branch/LConn1

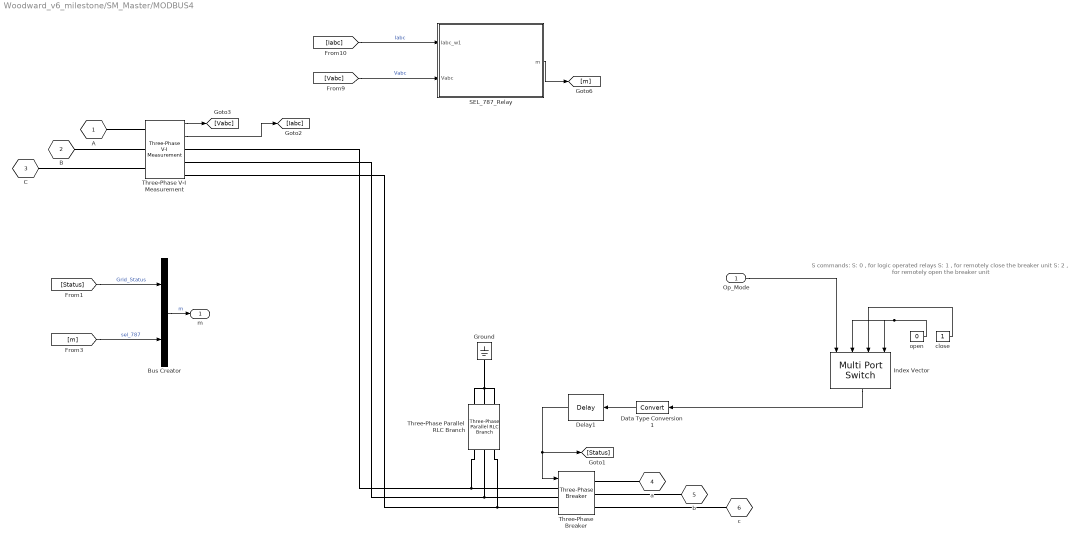
== system Woodward_v6_milestone/SM_Master/MODBUS4 ==
  note: S commands:
      | S: 0 , for logic operated relays
      | S: 1 ,  for remotely close the breaker unit
      | S: 2 , for remotely open the breaker unit
  Op_Mode : Inport
  Bus Creator : BusCreator  Inputs=2
  Data Type Conversion1 : DataTypeConversion
  Delay1 : dspsigops/Delay  dly_unit=Samples  delay=lower((3/60)/Ts)  ic_detail=off  dif_ic_for_ch=off  dif_ic_for_dly=off  ic=1  reset_popup=None
  Ground : powerlib/Elements/Ground  LConnTagsString=a
  Index Vector : MultiPortSwitch  DataPortOrder=Zero-based contiguous  DataPortIndices={2,1,0}  zeroidx=on
  SEL_787_Relay : Subsystem
  Three-Phase Parallel RLC Branch : powerlib/Elements/Three-Phase Parallel RLC Branch  LConnTagsString=A|B|C  RConnTagsString=A|B|C  BranchType=R  Resistance=10e6  Inductance=1e-3  Capacitance=1e-6  Measurements=None
  Three-Phase V-I Measurement : powerlib/Measurements/Three-Phase V-I Measurement  VoltageMeasurement=phase-to-ground  SetLabelV=off  LabelV=Vabc  Vpu=off  VpuLL=off  CurrentMeasurement=yes  SetLabelI=off  LabelI=Iabc  Ipu=off  Pbase=100e6  Vbase=500e3  OutputType=Complex  PhasorSimulation=off  PSBequivalent=0
  Three-Phase Breaker : powerlib/Elements/Three-Phase Breaker  InitialState=closed  SwitchA=on  SwitchB=on  SwitchC=on  SwitchTimes="[1/60  5/60]"  External=on  BreakerResistance=1e-3  SnubberResistance=0  SnubberCapacitance=0  Measurements=None
  close : Constant
  open : Constant  Value=0
  A : PMIOPort  Tag=PMCPort  Port=1  Side=Left
  B : PMIOPort  Tag=PMCPort  Port=2  Side=Left
  C : PMIOPort  Tag=PMCPort  Port=3  Side=Left
  a : PMIOPort  Tag=PMCPort  Port=4  Side=Right
  b : PMIOPort  Tag=PMCPort  Port=5  Side=Right
  c : PMIOPort  Tag=PMCPort  Port=6  Side=Right
  m : Outport
  wires:
  [m] -> Bus Creator/2  "sel_787"
  SEL_787_Relay/1(m) -> [m]
  Bus Creator/1 -> m/1  "m"
  [Status] -> Bus Creator/1  "Grid_Status"
  Delay1/1 -> [Status], Three-Phase Breaker/1
  Three-Phase V-I Measurement/1 -> [Vabc]
  Three-Phase V-I Measurement/2 -> [Iabc]
  open/1 -> Index Vector/4, Index Vector/2
  close/1 -> Index Vector/3
  Index Vector/1 -> Data Type Conversion1/1
  Data Type Conversion1/1 -> Delay1/1
  [Iabc] -> SEL_787_Relay/1(Iabc_w1)  "Iabc"
  [Vabc] -> SEL_787_Relay/2(Vabc)  "Vabc"
  Op_Mode/1 -> Index Vector/1
  connections:
  Three-Phase V-I Measurement/RConn1 -- Three-Phase Parallel RLC Branch/RConn1 -- Three-Phase Breaker/LConn1
  Three-Phase V-I Measurement/RConn2 -- Three-Phase Parallel RLC Branch/RConn2 -- Three-Phase Breaker/LConn2
  Three-Phase V-I Measurement/RConn3 -- Three-Phase Parallel RLC Branch/RConn3 -- Three-Phase Breaker/LConn3
  Three-Phase Breaker/RConn2 -- b/RConn1
  Three-Phase Breaker/RConn3 -- c/RConn1
  Three-Phase V-I Measurement/LConn1 -- A/RConn1
  a/RConn1 -- Three-Phase Breaker/RConn1
  C/RConn1 -- Three-Phase V-I Measurement/LConn3
  B/RConn1 -- Three-Phase V-I Measurement/LConn2
  Ground/LConn1 -- Three-Phase Parallel RLC Branch/LConn2 -- Three-Phase Parallel RLC Branch/LConn3 -- Three-Phase Parallel RLC Branch/LConn1

== system Woodward_v6_milestone/SM_Master/Test_load_2s ==
  In1 : Inport
  Constant Load : powerlib/Elements/Three-Phase Parallel RLC Load  LConnTagsString=A|B|C  Configuration=Y (grounded)  NominalVoltage=v  NominalFrequency=60  ActivePower=kVA*1E3*pf  InductivePower=kVA*1E3*sqrt(1-pf^2)  CapacitivePower=0  Measurements=None  LoadType=constant Z
  Constant Load1 : powerlib/Elements/Three-Phase Parallel RLC Load  LConnTagsString=A|B|C  Configuration=Y (grounded)  NominalVoltage=v  NominalFrequency=60  ActivePower=kVA*1E3*pf  InductivePower=kVA*1E3*sqrt(1-pf^2)  CapacitivePower=0  Measurements=None  LoadType=constant Z
  Three-Phase Breaker : powerlib/Elements/Three-Phase Breaker  InitialState=open  SwitchA=on  SwitchB=on  SwitchC=on  SwitchTimes=[15]  External=on  BreakerResistance=0.001  SnubberResistance=1e6  SnubberCapacitance=inf  Measurements=None
  A : PMIOPort  Port=1  Side=Left
  B : PMIOPort  Port=2  Side=Left
  C : PMIOPort  Port=3  Side=Left
  wires:
  In1/1 -> Three-Phase Breaker/1
  connections:
  A/RConn1 -- Constant Load/LConn1 -- Three-Phase Breaker/LConn1
  Three-Phase Breaker/LConn2 -- Constant Load/LConn2 -- B/RConn1
  Three-Phase Breaker/LConn3 -- Constant Load/LConn3 -- C/RConn1
  Constant Load1/LConn1 -- Three-Phase Breaker/RConn1
  Three-Phase Breaker/RConn2 -- Constant Load1/LConn2
  Constant Load1/LConn3 -- Three-Phase Breaker/RConn3

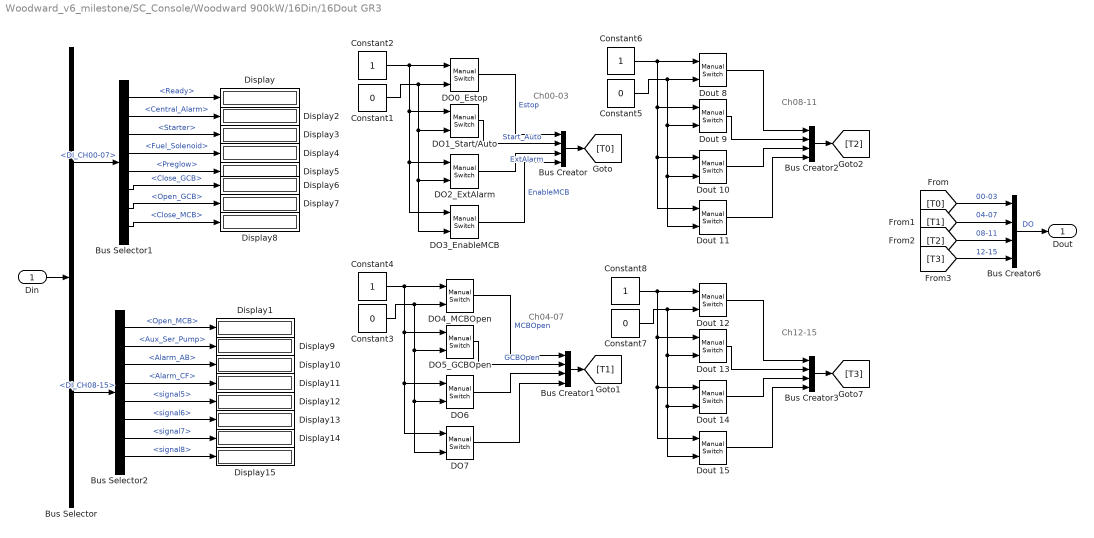
== system Woodward_v6_milestone/SC_Console/Woodward 900kW/16Din/16Dout GR3 ==
  note: Ch00-03
  note: Ch04-07
  note: Ch08-11
  note: Ch12-15
  Din : Inport
  Bus Creator{,1..3,6} (5 alike) : BusCreator
  Bus Selector : BusSelector  OutputSignals=DIN.DI_CH00-07,DIN.DI_CH08-15
  Bus Selector1 : BusSelector  OutputSignals=Ready,Central_Alarm,Starter,Fuel_Solenoid,Preglow,Close_GCB,Open_GCB,Close_MCB
  Bus Selector2 : BusSelector  OutputSignals=Open_MCB,Aux_Ser_Pump,Alarm_AB,Alarm_CF,signal5,signal6,signal7,signal8
  Constant{1,3,5,7} (4 alike) : Constant  Value=0
  Constant{2,4,6,8} (4 alike) : Constant
  DO0_Estop : simulink/Signal Routing/Manual Switch  sw=1  action=0  varsize=off
  DO1_Start/Auto : simulink/Signal Routing/Manual Switch  sw=0  action=0  varsize=off
  DO2_ExtAlarm : simulink/Signal Routing/Manual Switch  sw=0  action=0  varsize=off
  DO3_EnableMCB : simulink/Signal Routing/Manual Switch  sw=0  action=0  varsize=off
  DO4_MCBOpen : simulink/Signal Routing/Manual Switch  sw=0  action=0  varsize=off
  DO5_GCBOpen : simulink/Signal Routing/Manual Switch  sw=0  action=0  varsize=off
  DO6 : simulink/Signal Routing/Manual Switch  sw=0  action=0  varsize=off
  DO7 : simulink/Signal Routing/Manual Switch  sw=0  action=0  varsize=off
  Display{,1..15} (16 alike) : Display
  Dout {8..15} (8 alike) : simulink/Signal Routing/Manual Switch  sw=0  action=0  varsize=off
  Dout : Outport
  wires:
  Bus Creator6/1 -> Dout/1  "DO"
  Constant2/1 -> DO0_Estop/1, DO1_Start/Auto/1, DO3_EnableMCB/1, DO2_ExtAlarm/1
  Constant1/1 -> DO0_Estop/2, DO1_Start/Auto/2, DO3_EnableMCB/2, DO2_ExtAlarm/2
  DO0_Estop/1 -> Bus Creator/1  "Estop"
  DO1_Start/Auto/1 -> Bus Creator/2  "Start_Auto"
  DO2_ExtAlarm/1 -> Bus Creator/3  "ExtAlarm"
  DO3_EnableMCB/1 -> Bus Creator/4  "EnableMCB"
  Constant4/1 -> DO6/1, DO7/1, DO5_GCBOpen/1, DO4_MCBOpen/1
  Constant3/1 -> DO6/2, DO7/2, DO5_GCBOpen/2, DO4_MCBOpen/2
  DO4_MCBOpen/1 -> Bus Creator1/1  "MCBOpen"
  DO5_GCBOpen/1 -> Bus Creator1/2  "GCBOpen"
  DO6/1 -> Bus Creator1/3
  DO7/1 -> Bus Creator1/4
  Constant6/1 -> Dout 8/1, Dout 9/1, Dout 11/1, Dout 10/1
  Constant5/1 -> Dout 8/2, Dout 9/2, Dout 11/2, Dout 10/2
  Dout 8/1 -> Bus Creator2/1
  Dout 9/1 -> Bus Creator2/2
  Dout 10/1 -> Bus Creator2/3
  Dout 11/1 -> Bus Creator2/4
  Constant8/1 -> Dout 14/1, Dout 15/1, Dout 13/1, Dout 12/1
  Constant7/1 -> Dout 14/2, Dout 15/2, Dout 13/2, Dout 12/2
  Dout 12/1 -> Bus Creator3/1
  Dout 13/1 -> Bus Creator3/2
  Dout 14/1 -> Bus Creator3/3
  Dout 15/1 -> Bus Creator3/4
  Bus Creator/1 -> [T0]
  Bus Creator1/1 -> [T1]
  Bus Creator3/1 -> [T3]
  Bus Creator2/1 -> [T2]
  [T0] -> Bus Creator6/1  "00-03"
  [T1] -> Bus Creator6/2  "04-07"
  [T2] -> Bus Creator6/3  "08-11"
  [T3] -> Bus Creator6/4  "12-15"
  Din/1 -> Bus Selector/1
  Bus Selector/1 -> Bus Selector1/1  "<DI_CH00-07>"
  Bus Selector1/1 -> Display/1  "<Ready>"
  Bus Selector1/2 -> Display2/1  "<Central_Alarm>"
  Bus Selector1/3 -> Display3/1  "<Starter>"
  Bus Selector1/4 -> Display4/1  "<Fuel_Solenoid>"
  Bus Selector1/5 -> Display5/1  "<Preglow>"
  Bus Selector1/6 -> Display6/1  "<Close_GCB>"
  Bus Selector1/7 -> Display7/1  "<Open_GCB>"
  Bus Selector1/8 -> Display8/1  "<Close_MCB>"
  Bus Selector/2 -> Bus Selector2/1  "<DI_CH08-15>"
  Bus Selector2/1 -> Display1/1  "<Open_MCB>"
  Bus Selector2/2 -> Display9/1  "<Aux_Ser_Pump>"
  Bus Selector2/3 -> Display10/1  "<Alarm_AB>"
  Bus Selector2/4 -> Display11/1  "<Alarm_CF>"
  Bus Selector2/5 -> Display12/1  "<signal5>"
  Bus Selector2/6 -> Display13/1  "<signal6>"
  Bus Selector2/7 -> Display14/1  "<signal7>"
  Bus Selector2/8 -> Display15/1  "<signal8>"

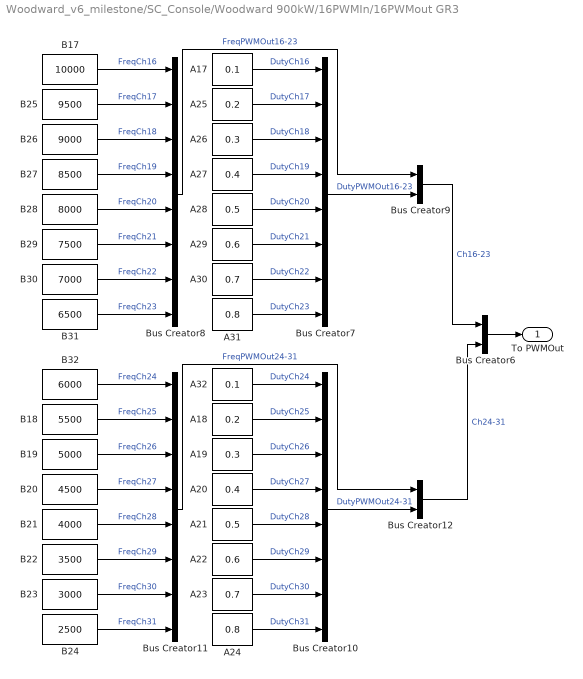
== system Woodward_v6_milestone/SC_Console/Woodward 900kW/16PWMIn/16PWMout GR3 ==
  A17 : Constant  Value=0.1
  A18 : Constant  Value=0.2
  A19 : Constant  Value=0.3
  A20 : Constant  Value=0.4
  A21 : Constant  Value=0.5
  A22 : Constant  Value=0.6
  A23 : Constant  Value=0.7
  A24 : Constant  Value=0.8
  A25 : Constant  Value=0.2
  A26 : Constant  Value=0.3
  A27 : Constant  Value=0.4
  A28 : Constant  Value=0.5
  A29 : Constant  Value=0.6
  A30 : Constant  Value=0.7
  A31 : Constant  Value=0.8
  A32 : Constant  Value=0.1
  B17 : Constant  Value=10000
  B18 : Constant  Value=5500
  B19 : Constant  Value=5000
  B20 : Constant  Value=4500
  B21 : Constant  Value=4000
  B22 : Constant  Value=3500
  B23 : Constant  Value=3000
  B24 : Constant  Value=2500
  B25 : Constant  Value=9500
  B26 : Constant  Value=9000
  B27 : Constant  Value=8500
  B28 : Constant  Value=8000
  B29 : Constant  Value=7500
  B30 : Constant  Value=7000
  B31 : Constant  Value=6500
  B32 : Constant  Value=6000
  Bus Creator{7..8,10..11} (4 alike) : BusCreator  Inputs=8
  Bus Creator12 : BusCreator  Inputs=2
  Bus Creator6 : BusCreator  Inputs=2
  Bus Creator9 : BusCreator  Inputs=2
  To PWMOut : Outport
  wires:
  Bus Creator6/1 -> To PWMOut/1
  A17/1 -> Bus Creator7/1  "DutyCh16"
  A25/1 -> Bus Creator7/2  "DutyCh17"
  A26/1 -> Bus Creator7/3  "DutyCh18"
  A27/1 -> Bus Creator7/4  "DutyCh19"
  A28/1 -> Bus Creator7/5  "DutyCh20"
  A29/1 -> Bus Creator7/6  "DutyCh21"
  A30/1 -> Bus Creator7/7  "DutyCh22"
  A31/1 -> Bus Creator7/8  "DutyCh23"
  B17/1 -> Bus Creator8/1  "FreqCh16"
  B25/1 -> Bus Creator8/2  "FreqCh17"
  B26/1 -> Bus Creator8/3  "FreqCh18"
  B27/1 -> Bus Creator8/4  "FreqCh19"
  B28/1 -> Bus Creator8/5  "FreqCh20"
  B29/1 -> Bus Creator8/6  "FreqCh21"
  B30/1 -> Bus Creator8/7  "FreqCh22"
  B31/1 -> Bus Creator8/8  "FreqCh23"
  Bus Creator7/1 -> Bus Creator9/2  "DutyPWMOut16-23"
  Bus Creator8/1 -> Bus Creator9/1  "FreqPWMOut16-23"
  A32/1 -> Bus Creator10/1  "DutyCh24"
  A18/1 -> Bus Creator10/2  "DutyCh25"
  A19/1 -> Bus Creator10/3  "DutyCh26"
  A20/1 -> Bus Creator10/4  "DutyCh27"
  A21/1 -> Bus Creator10/5  "DutyCh28"
  A22/1 -> Bus Creator10/6  "DutyCh29"
  A23/1 -> Bus Creator10/7  "DutyCh30"
  A24/1 -> Bus Creator10/8  "DutyCh31"
  B32/1 -> Bus Creator11/1  "FreqCh24"
  B18/1 -> Bus Creator11/2  "FreqCh25"
  B19/1 -> Bus Creator11/3  "FreqCh26"
  B20/1 -> Bus Creator11/4  "FreqCh27"
  B21/1 -> Bus Creator11/5  "FreqCh28"
  B22/1 -> Bus Creator11/6  "FreqCh29"
  B23/1 -> Bus Creator11/7  "FreqCh30"
  B24/1 -> Bus Creator11/8  "FreqCh31"
  Bus Creator10/1 -> Bus Creator12/2  "DutyPWMOut24-31"
  Bus Creator11/1 -> Bus Creator12/1  "FreqPWMOut24-31"
  Bus Creator12/1 -> Bus Creator6/2  "Ch24-31"
  Bus Creator9/1 -> Bus Creator6/1  "Ch16-23"

== system Woodward_v6_milestone/SC_Console/Woodward 900kW/16TSDIn/16 TSDOut GR3 ==
  Bus Creator1 : BusCreator  Inputs=3
  Din/Dout ch16-23 : Subsystem
  Din/Dout ch24-31 : Subsystem
  Dout state ctrl : Subsystem
  TSDout : Outport
  wires:
  Din/Dout ch24-31/1(Out1) -> Bus Creator1/2  "times CH24-31"
  Din/Dout ch16-23/1(Out1) -> Bus Creator1/1  "times CH16-23"
  Dout state ctrl/1(Event State OUT) -> Bus Creator1/3  "states"
  Bus Creator1/1 -> TSDout/1
